simulink model "Proj_9_part2"  (R2016a)
settings: Solver=ode4  StartTime=0.0  StopTime=0.6  FixedStep=0.001  RelTol=1e-3
undefined symbols (not defined in the file or in its folder): ess
settings Model: Creator=chok1124  LastModifiedBy=chok1124

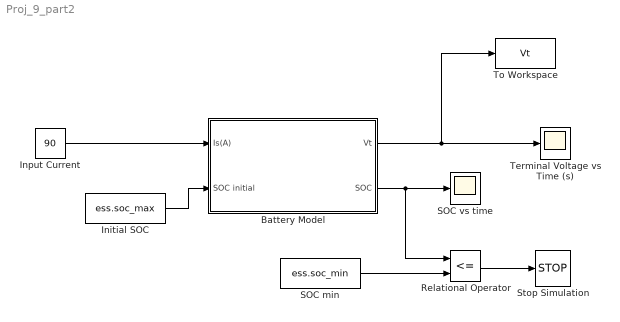
== system Proj_9_part2 ==
  Battery Model : Subsystem
  Initial SOC : Constant  Value=ess.soc_max
  Input Current : Constant  Value=90
  Relational Operator : RelationalOperator  Operator=<=  OutDataTypeStr=boolean
  SOC min : Constant  Value=ess.soc_min
  SOC vs time : Scope
  Stop Simulation : Stop
  Terminal Voltage vs Time (s) : Scope
  To Workspace : ToWorkspace  VariableName=Vt  SaveFormat=Timeseries  SampleTime=-1
  wires:
  Input Current/1 -> Battery Model/1(Is(A))
  Initial SOC/1 -> Battery Model/2(SOC initial)
  Battery Model/1(Vt) -> To Workspace/1, Terminal Voltage vs Time (s)/1
  Battery Model/2(SOC) -> Relational Operator/1, SOC vs time/1
  SOC min/1 -> Relational Operator/2
  Relational Operator/1 -> Stop Simulation/1

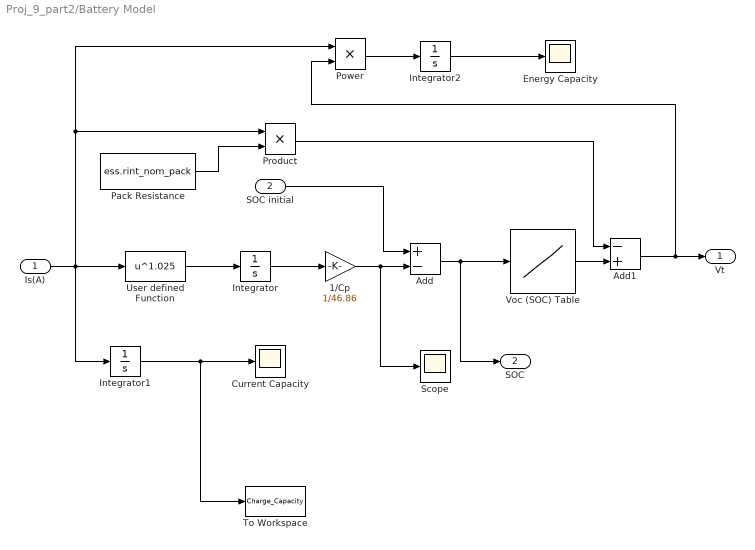
== system Proj_9_part2/Battery Model ==
  Is(A) : Inport
  SOC initial : Inport  Port=2
  1/Cp : Gain  Gain=1/46.86
  Add : Sum  Inputs=+-
  Add1 : Sum  Inputs=-+
  Current Capacity : Scope
  Energy Capacity : Scope
  Integrator : Integrator
  Integrator1 : Integrator
  Integrator2 : Integrator
  Pack Resistance : Constant  Value=ess.rint_nom_pack
  Power : Product
  Product : Product
  Scope : Scope
  To Workspace : ToWorkspace  VariableName=Charge_Capacity  SaveFormat=Timeseries  SampleTime=-1
  User defined Function : Fcn  Expr=u^1.025
  Voc (SOC) Table : Lookup_n-D  NumberOfTableDimensions=1  BreakpointsForDimension1=ess.soc_index  Table=ess.voc_map_pack  InternalRulePriority=Speed  RndMeth=Simplest  InputSameDT=on
  Vt : Outport
  SOC : Outport  Port=2
  wires:
  Integrator/1 -> 1/Cp/1
  Is(A)/1 -> Integrator1/1, User defined Function/1, Power/1, Product/1
  User defined Function/1 -> Integrator/1
  1/Cp/1 -> Scope/1, Add/2
  SOC initial/1 -> Add/1
  Pack Resistance/1 -> Product/2
  Product/1 -> Add1/1
  Add/1 -> SOC/1, Voc (SOC) Table/1
  Add1/1 -> Power/2, Vt/1
  Voc (SOC) Table/1 -> Add1/2
  Integrator1/1 -> To Workspace/1, Current Capacity/1
  Power/1 -> Integrator2/1
  Integrator2/1 -> Energy Capacity/1
